simulink model "MCU_vectorControl_with_fieldWeakening_dsPIC33CK_LVMC_FW_Hurst"  (R2018a)
settings: Solver=FixedStepDiscrete  StartTime=0.0  StopTime=10.0  FixedStep=50e-6  RelTol=1e-3  EnableMultiTasking=on
undefined symbols (not defined in the file): A0, A4, AN0, AN1, B0, B2, C12, C13, C14, C7, control, D11, D12, D13, D14, D5, D6, D7, DiscIntNeverNeededParam, inverter, Max, MaxPer, model, ms, NumBits1, NumBits2, P20, P32, P55, P60, P61, P62, P69, P70, P71, P75, P76, P77, P78, Pin, pmsm, PosRange1, PosRange2, PWM1max, Resol, s, Slope1, Slope2, us
libraries: simulink x45, MCHP_Blockset x23
(part 2 of 4)

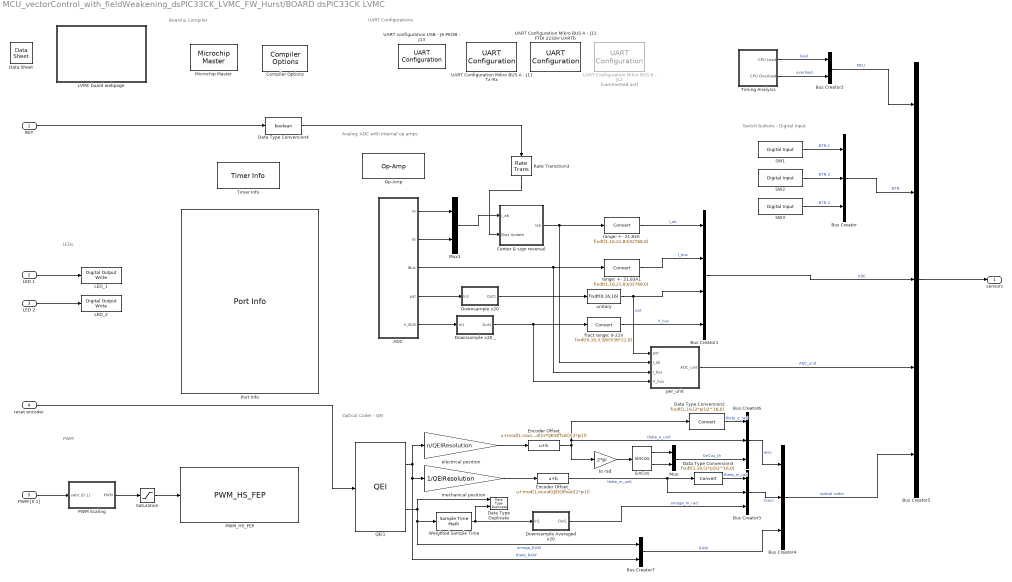
== system MCU_vectorControl_with_fieldWeakening_dsPIC33CK_LVMC_FW_Hurst/BOARD dsPIC33CK LVMC ==
  note: Board & Compiler
  note: Analog: ADC with internal op amps
  note: Optical Coder - QEI
  note: PWM
  note: UART Configurations
  note: LEDs
  note: Switch buttons - Digital Input
  INIT : Inport
  LED 1 : Inport  Port=2
  LED 2 : Inport  Port=3
  reset encoder : Inport  Port=4
  PWM [0 1] : Inport  Port=5  Unit=1
  ADC : Subsystem
  Bus Creator{,3..4,6} (4 alike) : BusCreator  Inputs=3
  Bus Creator1 : BusCreator  Inputs=4
  Bus Creator2 : BusCreator  Inputs=2
  Bus Creator5 : BusCreator  Inputs=5
  Bus Creator7 : BusCreator  Inputs=2
  Center & sign reversal : Subsystem
  Compiler Options : MCHP_Blockset/System Configuration/Compiler Options  Priority=1  LATEST_CMPLR=on  COMP_LIST=Dynamic Options  COMP_LIST_TXT=xc-dsc - v3.10  DFP_LIST=Dynamic Options  DFP_LIST_TXT=from compiler  CMSIS_DSP=Dynamic Options  CMSIS_DSP_TXT=Dynamic Options  USE_64BIT_DOUBLE=off  MCHP_MULTITHREAD_COMPILATION=on  UseCustom_LinkerScript=off  MCHP_MASTERLINK=MCU_vectorControl_with_fieldWeakening_dsPIC33CK_LVMC_FW_Hurst/BOARD dsPIC33CK LVMC/Microchip Master  OPTIMIZATION_LEVEL=2  MPLAB_LINKLIB=relaxed floating-point math  MPLAB_LINKLIB1=default  CodeReplacement=Dynamic Options  CodeReplacement_TXT=Microchip Code Replacement Library for dsPIC  OPTIMIZATION_FLTO=on  OPTIMIZATION_REORDER=off  UNROLL_LOOPS=off  PROCEDURAL_ABSTRACTION=off  GC_SECTIONS=None  MCODE=is more than 32768  MCONST=in code memory  MDATA=Can use all available memory  MSCALAR=Use only memory below address 8192 (faster)  MLARGEARRAY=off  MAGGREGATE=on  HEAP_SIZE=0  OMF=elf  DEBUG_INFO=on  ProduceHexOutput=on  AssemblyListing=off  SaveTemps=off  NO_EDS_WARN=on  PRINT_STATISTICS=off
      settings: SourceProductName=MPLAB Device Blocks for Simulink
  Data Sheet : MCHP_Blockset/System Info/Data Sheet  DOC_Type=datasheet  DOC_MCHP_Id=33FJ64MC802  DOC_FileLastCheckTime=[0 0 0 0 0 0]  cpy_MCHP_Id=33CK256MP508  MCHP_MASTERLINK=MCU_vectorControl_with_fieldWeakening_dsPIC33CK_LVMC_FW_Hurst/BOARD dsPIC33CK LVMC/Microchip Master
      settings: AttributesFormatString=%<cpy_MCHP_Id>  SourceProductName=MPLAB Device Blocks for Simulink
  Data Type Duplicate : DataTypeDuplicate
  Data Type Conversion2 : DataTypeConversion  OutDataTypeStr=fixdt(1,16,(2*pi)/2^16,0)  ConvertRealWorld=Stored Integer (SI)
  Data Type Conversion3 : DataTypeConversion  OutDataTypeStr=fixdt(1,16,(2*pi)/2^16,0)  ConvertRealWorld=Stored Integer (SI)
  Data Type Conversion4 : DataTypeConversion  OutDataTypeStr=boolean
  Downsample Averaged x20 : Subsystem  mask{DownSample=10}
      mask prompts: DownSample "DownSample Factor"
  Downsample x20 : Subsystem  mask{DownSample=20}
      mask prompts: DownSample "DownSample Factor"
  Downsample x20 _ : Subsystem  mask{DownSample=20}
      mask prompts: DownSample "DownSample Factor"
  Encoder Offset : Bias  Bias=mod(1,round((n*QEIOffset)/(2*pi)))
  Encoder Offset_ : Bias  Bias=mod(1,round(QEIOffset/(2*pi)))
  LED_1 : MCHP_Blockset/Digital IO/Digital Output Write  PORT=Dynamic Options  PORT_TXT="E   [ 0 : 15 ]"  PIN=6  PACK=off  SIMULTANEOUS=off  ORDERING=None  SampleTime=-1  MCHP_PORT={Digital Out}{DOU}1:1:E6;  MCHP_MASTERLINK=MCU_vectorControl_with_fieldWeakening_dsPIC33CK_LVMC_FW_Hurst/BOARD dsPIC33CK LVMC/Microchip Master
      settings: SourceProductName=MPLAB Device Blocks for Simulink
  LED_2 : MCHP_Blockset/Digital IO/Digital Output Write  PORT=Dynamic Options  PORT_TXT="E   [ 0 : 15 ]"  PIN=7  PACK=off  SIMULTANEOUS=off  ORDERING=None  SampleTime=-1  MCHP_PORT={Digital Out}{DOU}1:1:E7;  MCHP_MASTERLINK=MCU_vectorControl_with_fieldWeakening_dsPIC33CK_LVMC_FW_Hurst/BOARD dsPIC33CK LVMC/Microchip Master
      settings: SourceProductName=MPLAB Device Blocks for Simulink
  LVMC board webpage : Subsystem
      settings: OpenFcn=|
      | %web('www.microchip.com/DevelopmentTools/ProductDetails.aspx?PartNO=DM330021-2','-browser'); % MCLV2
      | web('https://www.microchip.com/en-us/development-tool/DM330031','-browser'); % LVMC
      | %pause(2);
      | %web('http://www.microchipdirect.com/productsearch.aspx?keywords=AC300020','-browser');
      | %web('www.microchipdirect.com/ProductSearch.aspx?keywords=AC300022','-browser');
      mask Display: image('MCHP_i_Board_LVMC_reduced.jpg');
  Microchip Master : MCHP_Blockset/System Configuration/Microchip Master  Priority=1  PICREF=33CK256MP508  TIMESTEP_REF=PWM1 Trigger 1 + ADC  BUSYFLAG=Dynamic Options  BUSYFLAG_TXT=None  VDD_range=Dynamic Options  PWRTEN=Not used  BOREN=Disable  BODENV=2.7V  BORV=Not used  FPWRT=128ms  DSBOREN=Enable ZPBOR during Deep Sleep Mode  DSLPBOR=Not used  MCLRE=Enabled  SMCLR=MCLR pin generates a normal system Reset  PMDL1WAY=Allow only one reconfiguration  RSTPRI=Device will obtain reset instruction from Primary flash  TEMP=Not used  SOSCSRC=Not used  SOSCSEL=Not used  IOL1WAY=Allow only one reconfiguration  ALTVREF=Not used  DISUVREG=Not used  DSSWEN=Not used  LPCFG=Not used  RTCBAT=Not used  VBTBOR=Not used  WUTSEL=Not used  POWERSAVE=off  ALTI2C=I2C mapped to SDA1/SCL1 pins  ALTI2C1=I2C1 mapped to SDA1/SCL1 pins  ALTI2C2=I2C2 mapped to SDA2/SCL2 pins  ALTI2C3=I2C3 mapped to SDA3/SCL3 pins  FDEVOPT1_ALTI2C1=Primary I2C1 pins are used  FDEVOPT1_ALTI2C2=Primary I2C2 pins are used  FDEVOPT1_SPI2MAPDIS=SPI2 pins are selected by peripheral pin selection feature  ALTQIO=QEA1; QEB1; INDX1 are selected as inputs to QEI1  ALTSS1=SS1A is selected as the I/O pin for SPI1  CMPPOL0=Hysteresis is applied to falling edge  CMPPOL1=Hysteresis is applied to falling edge  FCANIO=Not used  FETHIO=Default Ethernet I/O  FMIIEN=MII Enabled  FSRSSEL=Not used  FUSBIDIO=Controlled by the USB Module  FVBUSONIO=Not used  HPOL=PWM module high side output pins have active-high output polarity  HYST0=45 mV Hysteresis  HYST1=45 mV Hysteresis  I2C1SEL=Not used  LPOL=PWM module low side output pins have active-high output polarity  PWMPIN=PWM module pins controlled by PORT register at device Reset  RTCOSC=Not used  UPLLEN=USB PLL Disabled  UPLLIDIV=Not used  ATMOD8=Not used  ALTPMP=Not used  I2C2SEL=Not used  ALTADREF=Not used  ALTCVREF=Not used  PWMLOCK=PWM registers may be written without key sequence  INT_PRIORITY_DMA=0  MCHP_TIMER_RESULT=[ ]  MCHP_PLLRegisters="[1    100  16387     -1     33]"  MCHPVAR=MCHP.fcy.MIPS=1e+08;MCHP.fcy.SYSCLK=1e+08;MCHP.fcy.ADC=1e+08;MCHP.fcy.Comparator=1e+08;MCHP.fcy.I2C=1e+08;MCHP.fcy.SPI=1e+08;MCHP.fcy.UART=2e+08;MCHP.fcy.Timers=1e+08;MCHP.fcy.OC=1e+08;MCHP.fcy.IC=1e+08;MCHP.fcy.Ports=1e+08;MCHP.fcy.QEI=1e+08;MCHP.fcy.APLL=-1;MCHP.PowerSave=0;MCHP.TimeStepFactor=-20000;MCHP.TimeStep_Timer=-1;MCHP.NTIMERS=1;MCHP.id.name='33CK256MP508';MCHP.id.N=reshape([33 256 508],1,3);MCHP.id.L=reshape({ 'CK','MP',''},1,3);MCHP.id.Arch=3;MCHP.id.maskset='WACG';MCHP.id.dos='02949';MCHP.id.ds='70005349';MCHP.id.archTxt='33xxxx';MCHP.id.clonedfrom='DSPIC33CH128MP508';MCHP.id.isSlave=0;MCHP.id.isMaster=0;MCHP.periph.PPS.reg_RPINRx=reshape([-1 1 1 1 -1 1 1 1 1 1 1 1 1 1 1 1 1 1 1 1 1 1 -1 -1 1 1 1 1 1 1 1 1 1 1 1 1 1 1 1 1 1 1 1 -1 1 1 1 -1 -1 -1 -1 -1 1 -1 1 1 -1 -1 1 1 1 -1 -1 -1 -1 1 1 -1 -1 -1 -1 -1 -1 -1 -1 1 1 -1 -1 -1 -1 -1 -1 -1 1 1 1 1 1 1 1 -1 -1 -1 -1 -1 -1 1 1 1],1,100);MCHP.PPS.dsPIC.RP=reshape([-1 -1 -1 -1 -1 -1 -1 -1 -1 -1 -1 -1 -1 -1 -1 -1 -1 -1 -1 -1 -1 -1 -1 -1 -1 -1 -1 -1 -1 -1 -1 -1 16 17 18 19 20 21 22 23 24 25 26 27 28 29 30 31 32 33 34 35 36 37 38 39 40 41 42 43 44 45 46 47 48 49 50 51 52 53 54 55 56 57 58 59 60 61 62 63],1,80);MCHP.PPS.dsPIC.RPI=reshape(MCHP_Fun.Hex2num('[]'),0,0);MCHP.PPS.dsPIC.RPINR_list=reshape({ '1','INT1','INT2','INT3','5','T1CK','TCKI1','ICM1','TCKI2','ICM2','TCKI3','ICM3','TCKI4','ICM4','TCKI5','ICM5','TCKI6','ICM6','TCKI7','ICM7','TCKI8','ICM8','OCFA','OCFB','PCI8','PCI9','PCI10','PCI11','QEIA1','QEIB1','QEINDX1','QEIHOM1','QEIA2','QEIB2','QEINDX2','QEIHOM2','U1RX','U1DSR','U2RX','U2DSR','SDI1','SCK1_in','SS1_in','REFOI','SDI2','SCK2_in','SS2_in','48','QEIA3','QEIB3','QEINDX3','QEIHOM3','CAN1RX','CAN2RX','U3RX','U3DSR','57','58','SDI3','SCK3_in','SS3_in','CLCINE','CLCINF','CLCING','CLCINH','TCKI9','ICM9','68','69','70','71','72','73','74','OCFC','PCI17','PCI18','78','79','80','81','82','83','84','PCI12','PCI13','PCI14','PCI15','PCI16','SENT1','SENT2','CLCINA','CLCINB','CLCINC','CLCIND','ADCTRG','OCFD','U1CTS','U2CTS','U3CTS'},1,100);MCHP.PPS.dsPIC.RPOR_list=reshape({ '1','U1TX','U1RTS','U2TX','U2RTS','SDO1','SCK1_out','SS1_out','SDO2','SCK2_out','SS2_out','SDO3','SCK3_out','SS3_out','REFCLKO','OCM1','OCM2','OCM3','OCM4','OCM5','OCM6','CAN1TX','CAN2TX','CMP1','CMP2','CMP3','CMP4','U3TX','U3RTS','29','30','31','CMP5','CMP6','PWM4H','PWM4L','PWMEA','PWMEB','QEICCMP1','QEICCMP2','CLC1OUT','CLC2OUT','OCM7','OCM8','PWMEC','PWMED','PTGTRG24','PTGTRG25','SENT1OUT','SENT2OUT','MCCP9A','MCCP9B','MCCP9C','MCCP9D','MCCP9E','MCCP9F','56','57','58','CLC3OUT','CLC4OUT','U1DTR','U2DTR','U3DTR'},1,64);MCHP.PPS.dsPIC.RPV=reshape([176 177 178 179 180 181],1,6);MCHP.PPS.map_RPnR_RPORx=reshape([32 33 34 35 36 37 38 39 40 41 42 43 44 45 46 47 48 49 50 51 52 53 54 55 56 57 58 59 60 61 62 63 64 65 66 67 68 69 70 71 72 73 74 75 76 77 78 79 176 177 178 179 180 181],1,54);MCHP.Rx=reshape([16 34 15 74 2 -1 -1 -1 -1 -1 -1 18 35 28 73 4 -1 -1 -1 -1 -1 -1 20 41 29 72 17 -1 -1 -1 -1 -1 -1 21 43 33 69 19 -1 -1 -1 -1 -1 -1 23 45 63 68 22 -1 -1 -1 -1 -1 -1 -1 55 65 54 24 -1 -1 -1 -1 -1 -1 -1 56 30 53 37 -1 -1 -1 -1 -1 -1 -1 58 40 52 39 -1 -1 -1 -1 -1 -1 -1 60 46 49 42 -1 -1 -1 -1 -1 -1 -1 61 47 48 44 -1 -1 -1 -1 -1 -1 -1 75 66 38 57 -1 -1 -1 -1 -1 -1 -1 76 67 36 59 -1 -1 -1 -1 -1 -1 -1 78 5 27 62 -1 -1 -1 -1 -1 -1 -1 80 6 14 64 -1 -1 -1 -1 -1 -1 -1 1 7 13 77 -1 -1 -1 -1 -1 -1 -1 3 8 10 79 -1 -1 -1 -1 -1 -1],11,16);MCHP.ADC.ANtype=reshape([0 0],1,2);MCHP.ADC.ADCONx=reshape([0 0 0 0 0 0],1,6);MCHP.ADC.ADCHS_0=reshape([0 0],1,2);MCHP.ADC.Flags=reshape([-1 0],1,2);MCHP.ADC.Buffer=reshape([-1 -1],1,2);MCHP.ADC.port=reshape([0 18 23 3 4 16 17 18 19 2 24 25 32 33 34 35 39 38 58 59 64 65 66 67 -1 -1 -1 -1 -1 -1 -1 -1 -1 -1 -1 -1 -1 -1 -1 -1 -1 -1 -1 -1 -1 -1 -1 -1 -1 -1 -1 -1 -1 -1 -1 -1 -1],1,57);MCHP.ADC.port_ALT=reshape([-1 -1 -1 -1],1,4);MCHP.ADC.port_ALTA=reshape([18 1 -1 -1],1,4);MCHP.ADC.port_ALTB=reshape([-1 -1 -1 -1],1,4);MCHP.ADC.port_ALTC=reshape([-1 -1 -1 -1],1,4);MCHP.ADC.port_VrefP=-1;MCHP.ADC.port_VrefM=-1;MCHP.ADC.port_AVdd=-1;MCHP.ADC.port_AVss=-1;MCHP.ADC.ADCDATA=reshape([1 1 1 1 1 1 1 1 1 1 1 1 1 1 1 1 1 1 1 1 1 1 1 1 1 1 0 0 0 0 0 0 0 0 0 0 0 0 0 0 0 0 0 0 0 0 0 0 0 0 0 0 0 0 0 0 0],1,57);MCHP.ADC.HS_SAR.TRGSRC=reshape([1 1 1 1 1 1 1 1 1 1 1 1 1 1 1 1 1 1 1 1 1 1 1 1 1 1 0 0 0 0 0 0],1,32);MCHP.ADC.HS_SAR.nFilters=4;MCHP.ADC.HS_SAR.nDedicatedCore=2;MCHP.ADC.HS_SAR.CALIBRATION=0;MCHP.ADC.HS_SAR.ADCON1L=40960;MCHP.ADC.HS_SAR.ADC_Class3_idxStart=26;MCHP.memory.RAM=24576;MCHP.memory.RAM_XBegin=4096;MCHP.memory.RAM_YBegin=20480;MCHP.memory.RAM_dma=reshape([-1 -1],1,2);MCHP.memory.FLASH_ECC=0;MCHP.DMA.Num=4;MCHP.DMA.CNTmax=65535;MCHP.QEI.QEICONx=reshape([49023 49023 -1 -1 -1 -1],1,6);MCHP.QEI.QEItype=2;MCHP.QEI.Port_QEI_INDX=reshape([-1 -1],1,2);MCHP.QEI.Port_QEI_QEA=reshape([-1 -1],1,2);MCHP.QEI.Port_QEI_QEB=reshape([-1 -1],1,2);MCHP.QEI.Port_QEI_UPDN=reshape([-1 -1],1,2);MCHP.INT.Port=reshape([18 32767 32767 32767 -1],1,5);MCHP.ADC1.port=reshape([-1 -1 -1 -1 -1 -1 -1 -1 -1 -1 -1 -1 -1 -1 -1 -1 -1 -1 -1 -1 -1 -1 -1 -1 -1 -1 -1 -1 -1 -1 -1 -1],1,32);MCHP.ADC2.port=reshape([-1 -1 -1 -1 -1 -1 -1 -1 -1 -1 -1 -1 -1 -1 -1 -1 -1 -1 -1 -1 -1 -1 -1 -1 -1 -1 -1 -1 -1 -1 -1 -1],1,32);MCHP.ADC1N.port=reshape([-1 -1 -1 -1],1,4);MCHP.ADC2N.port=reshape([-1 -1 -1 -1],1,4);MCHP.PWM_HS.Flags=reshape([0 0 0],1,3);MCHP.PWM.port_FLT=reshape([-1 -1 -1 -1 -1 -1 -1 -1 -1 -1 -1 -1 -1 -1 -1 -1 -1 -1 -1 -1 -1 -1 -1 -1 -1 -1 -1 -1 -1 -1 -1 -1 -1],1,33);MCHP.PWM.PWMRef=-1;MCHP.PWM.Flag=0;MCHP.PWM.Port_PWM_l=reshape([31 -1 29 -1 27 -1 48 -1 37 -1 47 -1 43 -1 45 -1 -1 -1 -1 -1 -1 -1 -1 -1],2,12);MCHP.PWM.Port_PWM_h=reshape([30 -1 28 -1 26 -1 49 -1 36 -1 46 -1 42 -1 44 -1 -1 -1 -1 -1 -1 -1 -1 -1],2,12);MCHP.PWM_HS_FEP.nEVTOUT=5;MCHP.IC.Port=reshape([0 0 0 0 0 0 0 0 0 0 0 0 0 0 0 0],1,16);MCHP.IC.type=-1;MCHP.OC.Port=reshape([0 0 0 0 0 0 0 0 0 0 0 0 0 0 0 0],1,16);MCHP.OC.type=-1;MCHP.CN.Port=reshape([-1 -1 -1 -1 -1 -1 -1 -1 -1 -1 -1 -1 -1 -1 -1 -1 -1 -1 -1 -1 -1 -1 -1 -1 -1 -1 -1 -1 -1 -1 -1 -1 -1 -1 -1 -1 -1 -1 -1 -1 -1 -1 -1 -1 -1 -1 -1 -1 -1 -1 -1 -1 -1 -1 -1 -1 -1 -1 -1 -1 -1 -1 -1 -1 -1 -1 -1 -1 -1 -1 -1 -1 -1 -1 -1 -1 -1 -1 -1 -1 -1 -1 -1 -1 -1],1,85);MCHP.CN.PullUp=reshape([31 65535 65535 65535 65535 0 0 0 0 0 0],1,11);MCHP.CN.type=2;MCHP.CN.Flag_PullDown=1;MCHP.SPI.Refs=reshape([1 2 3 0 0 0],1,6);MCHP.SPI.SPIxCON1=-1;MCHP.SPI.SPIxCON2=-1;MCHP.SPI.SPIxFIFOSIZE=4;MCHP.SPI.Port_SDI=reshape([-1 41 -1 -1 -1 -1],1,6);MCHP.SPI.Port_SDO=reshape([-1 56 -1 -1 -1 -1],1,6);MCHP.SPI.Port_SCK=reshape([-1 40 -1 -1 -1 -1],1,6);MCHP.SPI.Port_SS=reshape([-1 -1 -1 -1 -1 -1],1,6);MCHP.I2C.Refs=reshape([1 2 3 0 0],1,5);MCHP.I2C.I2CxCON=49151;MCHP.I2C.NewRegName=2;MCHP.I2C.Port_SDA=reshape([25 21 23 -1 -1],1,5);MCHP.I2C.Port_SCL=reshape([24 22 18 -1 -1],1,5);MCHP.I2C.Port_ASDA=reshape([40 36 52 -1 -1],1,5);MCHP.I2C.Port_ASCL=reshape([41 37 51 -1 -1],1,5);MCHP.I2C.Fuse_Port_SCL_SDA=reshape([29 1 30 1 31 1 -1 -1 -1 -1],2,5);MCHP.I2C.Fuse_Port_ASCL_ASDA=reshape([29 2 30 2 31 2 -1 -1 -1 -1],2,5);MCHP.SCCP.nSCCP=9;MCHP.SCCP.MCCP=reshape([0 0 0 0 0 0 0 0 0],1,9);MCHP.PGA.Port_PGA1P=reshape([-1 -1 -1 -1],1,4);MCHP.PGA.Port_PGA1N=reshape([-1 -1 -1 -1],1,4);MCHP.PGA.Port_PGA2P=reshape([-1 -1 -1 -1],1,4);MCHP.PGA.Port_PGA2N=reshape([-1 -1 -1 -1],1,4);MCHP.PGA.Num=0;MCHP.HS_AnalogComparator.Port_CMP1=reshape([0 33 3 18],1,4);MCHP.HS_AnalogComparator.Port_CMP2=reshape([35 34 59 18],1,4);MCHP.HS_AnalogComparator.Port_CMP3=reshape([23 4 58 18],1,4);MCHP.HS_AnalogComparator.Port_CMP4=reshape([-1 -1 -1 -1],1,4);MCHP.HS_AnalogComparator.PORT_EXTREFx=reshape([-1 -1],1,2);MCHP.HS_AnalogComparator.Port_DACOUTx=reshape([3 -1],1,2);MCHP.HS_AnalogComparator.Num=0;MCHP.Comp.Port_CVrefin=-1;MCHP.Comp.Port_CVref=-1;MCHP.Comp.Port_CVref1O=-1;MCHP.Comp.Port_CVref2O=-1;MCHP.Comp.Port_CxOUT=reshape([32767 32767 32767 32767 32767],1,5);MCHP.Comp.Port_OAxOUT=reshape([0 18 4 -1 -1],1,5);MCHP.Comp.Port_CxINP=reshape([-1 -1 -1 -1 -1],1,5);MCHP.Comp.Port_CxINM=reshape([-1 -1 -1 -1 -1 -1 -1 -1 -1 -1 -1 -1 -1 -1 -1 -1 -1 -1 -1 -1],4,5);MCHP.Comp.Port_OAxINP=reshape([2 20 34 -1 -1],1,5);MCHP.Comp.Port_OAxINM=reshape([1 19 33 -1 -1],1,5);MCHP.Comp.nComp=reshape([5 0 0],1,3);MCHP.Comp.OpAmp=0;MCHP.Comp.CVRCON=reshape([0 0],1,2);MCHP.Comp.CMCON=0;MCHP.CDAC.Port_DACx=reshape([-1 -1 -1],1,3);MCHP.CDAC.nCDAC=0;MCHP.UART.port_Rx=reshape([32767 32767 32767 -1 -1 -1],1,6);MCHP.UART.port_Tx=reshape([32767 32767 32767 -1 -1 -1],1,6);MCHP.UART.port_ARx=reshape([-1 -1],1,2);MCHP.UART.port_ATx=reshape([-1 -1],1,2);MCHP.UART.port_RTS=reshape([32767 32767 32767 -1 -1 -1],1,6);MCHP.UART.port_CTS=reshape([32767 32767 32767 -1 -1 -1],1,6);MCHP.UART.reg_UxMODE=reshape([48127 48127 48127 -1 -1 -1],1,6);MCHP.UART.reg_UxSTA=reshape([65535 65535 65535 -1 -1 -1],1,6);MCHP.modsrc.DOS_04094_cpu_33a_v1_dspic33a=0;MCHP.modsrc.DOS_04436_perseus_dspic33a=0;MCHP.modsrc.DOS_04928_gpio_ports_upb_v2_dspic33a=0;MCHP.modsrc.DOS_02672_math_progcrc_upb_v1_dspic33a=0;MCHP.modsrc.DOS_04993_sec_32bit_cp_upb_v1_dspic33a=0;MCHP.modsrc.DOS_03681_bmx_33a_upb_v1_dspic33a=0;MCHP.modsrc.DOS_03459_adc_pc_ctrl_upb_v2_dspic33a=0;MCHP.modsrc.DOS_04302_pwm_pc_upb_v3_dspic33a=0;MCHP.modsrc.DOS_03076_uart_protocol_upb_v1_dspic33a=0;MCHP.modsrc.DOS_01482_spi_i2s_upb_v1_dspic33a=0;MCHP.modsrc.DOS_05155_i2c_upb_v4_dspic33a=0;MCHP.modsrc.DOS_02359_sent_j2716_upb_v1_dspic33a=0;MCHP.modsrc.DOS_05177_qei_32b_upb_v2_dspic33a=0;MCHP.modsrc.DOS_01512_ccp_mccp_upb_v1_dspic33a=0;MCHP.modsrc.DOS_03496_dac_pdm_nbit_upb_v2_dspic33a=0;MCHP.modsrc.DOS_02673_tmr_classa_upb_v1_dspic33a=0;MCHP.modsrc.DOS_04776_perf_mon_upb_v1_dspic33a=0;MCHP.modsrc.DOS_03680_pfm_pbu_33a_upb_v1_dspic33a=0;MCHP.modsrc.DOS_04649_sec_pac_upb_v0_dspic33a=0;MCHP.modsrc.DOS_03966_io_integrity_monitor_upb_v1_dspic33a=0;MCHP.modsrc.DOS_04641_biss_master_upb_v1_dspic33a=0;MCHP.modsrc.DOS_04077_dma_upb_v1_dspic33a=0;MCHP.modsrc.DOS_04549_nvm_ctrl_32bit_upb_v1_dspic33a=0;MCHP.modsrc.DOS_04449_clk_cru_33a_upb_v1_dspic33a=0;MCHP.modsrc.DOS_03850_clk_monitor_upb_v1_dspic33a=0;MCHP.modsrc.DOS_04342_osc_rc8mhz_ctrl_upb_v4_dspic33a=0;MCHP.modsrc.DOS_04650_wdt_upb_v4_dspic33a=0;MCHP.modsrc.DOS_05178_ptg_pc_upb_v1_dspic33a=0;MCHP.modsrc.DOS_04181_data_ram_ctrl_upb_v1_dspic33a=0;MCHP.modsrc.DOS_04735_wdt_dmt_upb_v6_dspic33a=0;MCHP.modsrc.DOS_01577_cla_clc_upb_v1_dspic33a=0;MCHP.modsrc.DOS_03516_pwr_sib_upb_v3_dspic33a=0;MCHP.modsrc.DOS_03495_amp_pad_opamp_ctrl_upb_v2_dspic33a=0;MCHP.modsrc.DOS_05308_pegasus_dspic33a=0;MCHP.modsrc.DOS_02976_adc_12b_upb_v2_dspic33a=0;MCHP.modsrc.DOS_05404_adc_pc_ctrl_upb_v3_dspic33a=0;MCHP.modsrc.DOS_05226_pwm_pc_upb_v4_dspic33a=0;MCHP.modsrc.DOS_05226_apwm_pc_upb_v4_dspic33a=0;MCHP.modsrc.DOS_05431_dac_pdm_nbit_upb_v3_dspic33a=0;MCHP.modsrc.DOS_04649_sec_pac_upb_v1_dspic33a=0;MCHP.modsrc.DOS_05461_pwr_sib_upb_v4_dspic33a=0;MCHP.modsrc.DOS_05420_amp_vref_ctl_upb_v1_dspic33a=0;MCHP.modsrc.DOS_03267_adc_soft_code_seq_v1_dspic33a=0;MCHP.modsrc.DOS_04537_can_fd_upb_v3_dspic33a=0;MCHP.modsrc.DOS_05346_sec_cam_lite_v2_dspic33a=0;MCHP.modsrc.DOS_02551_cpu_16bit_v7=1;MCHP.modsrc.DOS_01520_wdt_dmt_upb_v1_16bit=1;MCHP.modsrc.DOS_02359a_sent_j2716_upb_v1=1;MCHP.modsrc.DOS_02672_math_progcrc_upb_v1_16bit=1;MCHP.modsrc.DOS_01577_cla_clc_upb_v1=1;MCHP.modsrc.DOS_02915_ecc_v2=1;MCHP.modsrc.DOS_02673_tmr_classa_upb_v1_16bit=1;MCHP.modsrc.DOS_01494_qei_32b_upb_v1_16bit=1;MCHP.modsrc.DOS_02472_ppi_pmp16_upb_v1_16bit=1;MCHP.modsrc.DOS_01441_i2c_upb_v1_16bit_TLAH=1;MCHP.modsrc.DOS_03076_uart_protocol_upb_v1_16bit=1;MCHP.modsrc.DOS_01482=1;MCHP.modsrc.DOS_01483_pwm_16bit=1;MCHP.modsrc.DOS_03247_CAN_FD_UPB_V2_16_bit=1;MCHP.modsrc.DOS_02949_WACG=1;MCHP.modsrc.DOS_02316_nvm_ctrl_v1_16bit=1;MCHP.modsrc.DOS_03349_amp_pad_opamp_ctrl_upb_v1=1;MCHP.modsrc.DOS_02653_afe_current_bias_ctrl_upb_v1_16bit=1;MCHP.modsrc.DOS_01459_ptg_pc_upb_v1_16bit=1;MCHP.modsrc.DOS_01512_ccp_mccp_upb_v1_16bit=1;MCHP.modsrc.DOS_02519_dma_sfr_16bit_v2=1;MCHP.modsrc.DOS_02508c11=1;MCHP.modsrc.DOS_02475_dac_pdm_nbit_upb_v1_16bit=1;MCHP.modsrc.DOS_02467_gpio_upb_v1_16bit=1;MCHP.modsrc.DOS_00805_rst_integration_v4=1;MCHP.modsrc.DOS_02659_clk_sib_v12=1;MCHP.modsrc.DOS_02237_osc_dco_ctrl_upb_v1_16bit=1;MCHP.modsrc.DOS_02674_wdt_upb_v1_16bit=1;MCHP.modsrc.DOS_01407=1;MCHP.modsrc.DOS_03994_WAC07=0;MCHP.modsrc.DOS_02552_msi_upb_v1_Master=0;MCHP.modsrc.DOS_03667_pwm_pc_upb_v2_16bit=0;MCHP.modsrc.DOS_04180_drm_ctrl_ecc_v1=0;MCHP.modsrc.DOS_03431_STX03=0;MCHP.modsrc.DOS_03516_pwr_sib_upb_v3=0;MCHP.modsrc.DOS_02552_msi_upb_v1_Slave=0;MCHP.modsrc.DOS_04621_amp_pga_ctrl_upb_v3=0;MCHP.modsrc.DOS_02497_WACV=0;MCHP.modsrc.DOS_02593_amp_pga_ctrl_pb_v2_16bit=0;MCHP.modsrc.DOS_01461_afe_ctmu_con_upb_v1_16bit=0;MCHP.modsrc.DOS_02497_WACA=0;MCHP.modsrc.DOS_02478_uart_irda_upb_v1_16bit=0;MCHP.modsrc.DOS_00929=0;MCHP.modsrc.DOS_01198=0;MCHP.modsrc.DOS_03029_WACH=0;MCHP.modsrc.DOS_01483_apwm_16bit=0;MCHP.modsrc.DOS_04797_WAC0A=0;MCHP.modsrc.DOS_04884_WAC0B=0;MCHP.modsrc.DOS_04797_WAC09=0;MCHP.modsrc.DOS_03662_WACU=0;MCHP.modsrc.DOS_00794=0;MCHP.modsrc.DOS_00931=0;MCHP.modsrc.DOS_00932=0;MCHP.modsrc.DOS_00942=0;MCHP.modsrc.DOS_00938=0;MCHP.modsrc.DOS_00996=0;MCHP.modsrc.DOS_00997=0;MCHP.modsrc.DOS_00998=0;MCHP.modsrc.DOS_00209=0;MCHP.modsrc.DOS_01555_adc=0;MCHP.modsrc.DOS_01293=0;MCHP.modsrc.DOS_00828=0;MCHP.modsrc.DOS_01116=0;MCHP.modsrc.DOS_01017_RPORx=0;MCHP.modsrc.DOS_01017_RPINRx=0;MCHP.modsrc.DOS_01555_nvm_tsmc18_v2_16bit=0;MCHP.modsrc.DOS_00804=0;MCHP.modsrc.DOS_00826=0;MCHP.modsrc.DOS_01555_TLAK_PMDx=0;MCHP.modsrc.DOS_01555_TLAK_INT_=0;MCHP.modsrc.DOS_00933=0;MCHP.modsrc.DOS_01555=0;MCHP.modsrc.DOS_01555_ptg=0;MCHP.modsrc.DOS_00958=0;MCHP.modsrc.DOS_01117_PORTx=0;MCHP.modsrc.DOS_00999=0;MCHP.modsrc.DOS_01041=0;MCHP.modsrc.DOS_00892=0;MCHP.modsrc.DOS_01287_TLAC_PMDx=0;MCHP.modsrc.DOS_01287_TLAC_INT_=0;MCHP.modsrc.DOS_01424=0;MCHP.modsrc.DOS_01332=0;MCHP.modsrc.DOS_01468_PMBA_current_source=0;MCHP.modsrc.DOS_02291_PGA=0;MCHP.modsrc.DOS_01467_Comparator=0;MCHP.modsrc.DOS_01498_TLAY=0;MCHP.modsrc.DOS_00993_PLL_120MHz=0;MCHP.modsrc.DOS_01332_ptg_pc_v1=0;MCHP.modsrc.DOS_00958_pwm_TLAY=0;MCHP.modsrc.TLAY_IOPorts=0;MCHP.modsrc.DOS_00929q=0;MCHP.modsrc.DOS_02415_spi_v5=0;MCHP.modsrc.DOS_RPINRx_16bit_2=0;MCHP.modsrc.DOS_01497_TLAH_PMDx=0;MCHP.modsrc.DOS_02550_TLAL_INT=0;MCHP.modsrc.DOS_00958_pwm_TLAH=0;MCHP.modsrc.DOS_01287_TLAH_INT_=0;MCHP.modsrc.DOS_01113=0;MCHP.modsrc.DOS_01017_PMDx=0;MCHP.modsrc.DOS_00927=0;MCHP.modsrc.DOS_01080=0;MCHP.modsrc.DOS_00794_cpu_16bit_v3=0;MCHP.modsrc.DOS_02192_TLCD_PMDx=0;MCHP.modsrc.DOS_02192_TLCD_INT_=0;MCHP.modsrc.DOS_02192_cmp=0;MCHP.modsrc.DOS_00958_pwm_TLCD=0;MCHP.modsrc.DOS_02192_PORTx_TLCD=0;MCHP.modsrc.DOS_00936=0;MCHP.modsrc.DOS_00995=0;MCHP.modsrc.DOS_00546=0;MCHP.modsrc.DOS_00474=0;MCHP.modsrc.DOS_02481_WACK_MC_Config=0;MCHP.modsrc.DOS_03088_pfm_cache_ocp_v2_WACK=0;MCHP.modsrc.DOS_02819_pfm_ctrl_32bit_upb_v2=0;MCHP.modsrc.DOS_02674_wdt_upb_v1_32bit=0;MCHP.modsrc.DOS_01520_wdt_dmt_upb_v1=0;MCHP.modsrc.DOS_02869_icd_jtag_bvci_upb_v2=0;MCHP.modsrc.DOS_02823_WACJ_clk_cru_upb_v2=0;MCHP.modsrc.DOS_02823_WACN_clk_cru_upb_v2=0;MCHP.modsrc.DOS_01423_RPINRx=0;MCHP.modsrc.DOS_02481_RPORx=0;MCHP.modsrc.DOS_02511_pwr_sib_upb_v1_32bit=0;MCHP.modsrc.DOS_02907_WACN_GP_int_evic_v3=0;MCHP.modsrc.DOS_01500_dma_bvci_v2=0;MCHP.modsrc.DOS_02141_tmr_classa_pb_v2=0;MCHP.modsrc.DOS_02815_tmr_classb_upb_v1=0;MCHP.modsrc.DOS_00740_icap_pb_v1=0;MCHP.modsrc.DOS_00749_ocmp_pb_v1=0;MCHP.modsrc.DOS_01441_i2c_upb_v1_32bit=0;MCHP.modsrc.DOS_01329_spi_pb_v2=0;MCHP.modsrc.DOS_02478_uart_irda_upb_v1_32bit=0;MCHP.modsrc.DOS_03554_cmp_control_upb_v2_32bit=0;MCHP.modsrc.DOS_01445_dac_nbit__control_upb_v1_32bit=0;MCHP.modsrc.DOS_01461_afe_ctmu_con_upb_v1=0;MCHP.modsrc.DOS_01577_cla_clc_upb_v1_32bit=0;MCHP.modsrc.DOS_02467_gpio_ports_upb_v1=0;MCHP.modsrc.DOS_02508_adc_sar_ctrl_upb_v1_PIC32MK=0;MCHP.modsrc.DOS_01261_tmr_rtcc_pb_v2=0;MCHP.modsrc.DOS_01475_lpwr_deep_sleep_ctrl_v2=0;MCHP.modsrc.DOS_EIP_00136_ssx_v1=0;MCHP.modsrc.DOS_02907_WACN_MC_int_evic_v3=0;MCHP.modsrc.DOS_01477_pwm_mc_upb_v1=0;MCHP.modsrc.DOS_01494_qei_32b_upb_v1=0;MCHP.modsrc.DOS_03247_can_fd_upb_v2_pic32mk=0;MCHP.modsrc.DOS_02907_WACK_MC_int_evic_v3=0;MCHP.modsrc.DOS_02514_dfm_strl_sst_upb_v1=0;MCHP.modsrc.DOS_02472_ppi_pmp16_upb_v1=0;MCHP.modsrc.DOS_02813a_usb_otgcore_pb_v3=0;MCHP.modsrc.DOS_02481_WACJ_MC_Config=0;MCHP.modsrc.DOS_02569_pfm_cache_ocp_v1=0;MCHP.modsrc.DOS_02481_WACJ_MC_int_evic_v3=0;MCHP.modsrc.DOS_01459_ptg_pc_upb_v1_SIC=0;MCHP.modsrc.DOS_01427_cmp_control_upb_v1_32bit=0;MCHP.modsrc.DOS_01152_can_bvci_v1=0;MCHP.modsrc.DOS_02787_WACD_Config=0;MCHP.modsrc.DOS_00800_dac_4bit_ctrl_pb_v1=0;MCHP.modsrc.DOS_01539_icd_jtag_pb_v2=0;MCHP.modsrc.DOS_02823_clk_cru_upb_v2=0;MCHP.modsrc.DOS_01423_RPORx=0;MCHP.modsrc.DOS_02907_WACD_int_evic_v3=0;MCHP.modsrc.DOS_00734_uart_irda_pb_v1=0;MCHP.modsrc.DOS_00687_tmr_classa_pb_v1=0;MCHP.modsrc.DOS_00745_tmr_classb_pb_v1=0;MCHP.modsrc.DOS_02508_adc_sar_ctrl_upb_v1=0;MCHP.modsrc.DOS_00866_cmp_control_pb_v2=0;MCHP.modsrc.DOS_01114_eth_bvci_v1=0;MCHP.modsrc.DOS_02831_usb_clk_rst_v2=0;MCHP.modsrc.DOS_01643_pfm_cache_ahb_v2=0;MCHP.modsrc.DOS_EIP_00206r5_sqi_v2=0;MCHP.modsrc.DOS_EIP_00124_usb_hs_otgcore_v1=0;MCHP.modsrc.DOS_EIP_00218_math_rng_ahbs_v2=0;MCHP.modsrc.DOS_EIP_00109_ebi_v1=0;MCHP.modsrc.DOS_EIP_00158_crypto_v1=0;MCHP.PortBase=16;MCHP.PortPrefixe='P';MCHP.clock.PBxDIV=-1;MCHP.clock.CLKx_INTDIV=reshape([-1 -1 -1 -1 -1 -1 -1 -1 -1 -1 -1 -1 -1],1,13);MCHP.clock.CLKx_FRACDIV=reshape([-1 -1 -1 -1 -1 -1 -1 -1 -1 -1 -1 -1 -1],1,13);  MCHP_CRC=19007516  BTMODE=Device is in Single Boot (legacy) mode  RES1=Not used  RES2=Not used  ALTCMPI=Not used  BOREN1=Not used  ALTRB6=Not used  WDTEN=Disable  DBCC=No Cross Connection between DAC outputs  BOREN0=Enabled  DMTIVT=Not used  DMTCNT=2^31 (2147483648)  DMTEN=Dead Man Timer is Disabled and can be enabled by software  ON=Not used  USERID=Not used  RESERVED1=Not used  DMTINTV=Window/Interval value is 127/128 counter value  WDTSPGM=WDT stops during Flash programming  FDMTEN=Deadman Timer is disabled  BOOTISA=Boot code and Exception code is MIPS32  FSLEEP=Flash is powered down when the device is in Sleep mode  TSEQ=Not used  CSEQ=Not used  BORLVL=BOR trip point is 2.96 V  BSSO=Normal startup operation after reset; execute instruction at 0x000000  MCA=Flash read accesses are 2 cycle to support maximum processor frequency of operation  MAXTEMP=20 ns flash access  CFGAN14=Device pin is input to AN14  CFGAN15=Device pin is input to AN15  BISTDIS=mBIST on reset feature disabled  NOBTSWP=BOOTSWP instruction is disabled  BSEQ=Not used  IBSEQ=Not used  SMB3EN=SMBus 3.0 input levels  FUSBIDIO2=USBID pin is controlled by the USB2 module  FVBUSIO2=VBUSON pin is controlled by the USB2 module  FUSBIDIO1=USBID pin is controlled by the USB1 module  FVBUSIO1=VBUSON pin is controlled by the USB1 module  VBATBOREN=Enable ZPBOR during VBAT Mode  FDSEN=Enable DSEN bit in DSCON  BORSEL=BOR trip voltage 2.1v (Non-OPAMP deviced operation)  POSCFGAIN=Gain is G3  POSCAGCDLY=Settling time = 25ms x AGCRNG  POSCAGCRNG=Range 1x  POSCAGC=Automatic Gain Control for Oscillator  FDBGWP=Not used  FNOSC=Internal Fast RC (FRC)  FPR=ECIO w/ PLL 16x  FOSFPR=HS3 w/PLL 16x  FOS=Primary Oscillator  FRANGE=High Range  OSCILLATOR_SELECT=Internal Fast RC (FRC)  OSCILLATOR_SELECT_spd=Internal Fast RC (FRC)  QUARTZ=8e6  QUARTZ_spd=8e6  POSCGAIN=2x gain setting  POSCBOOST=Boost the kick start of the oscillator  SOSCGAIN=2x gain setting  SOSCBOOST=Boost the kick start of the oscillator  ACTIV_PLL=on  ACTIV_PLL_spd=on  MIPS_DESIRED=100e6  MIPS_DESIRED_spd=100e6  CPUDIV=Divide by 1  FPLLMUL=Not used  FPLLIDIV=8x Divider  POSCFREQ=Not used  POSCMD=Primary Oscillator Disabled  POSCMOD=Primary Oscillator Disabled  MIPS=100 * 1e6  ACLKCON=Optimized for PWM resolution & ADC conversion speed  ACLKCON_spd=Optimized for PWM resolution & ADC conversion speed  FPLLODIV=32x Divider  PLLKEN=PLL lock signal will be used to disable PLL clock output if lock is lost  FCKSM=Clock switching is enabled;Fail-safe Clock Monitor is disabled  FCKSMEN=Sw Disabled; Mon Disabled  IESO=Start up with FRC; then switch  DSWDTPS=1:2^36  FWDTEN=WDT controlled via SW; use WDTCON.ON bit  FWDTWINSZ=Window size is 25%  FWPSA=1:512  FWPSA0=1:128  FWPSB=1:16  WDT=Disable  WDTPOST=1:32768  WDTPRE=1:128  WDTPS=1:32768  WINDIS=Watchdog Timer operates in Non-Window mode  WWDTEN=Non-Window mode  DSWDTEN=Enable DSWDT during Deep Sleep Mode  DSWDTOSC=Select LPRC as DSWDT Reference clock  FWDT_RCLKSEL=WDT Run Mode uses BFRC:256  FWDT_RWDTPS=1:2147483648  FWDT_SWDTMPS=1:2147483648  FWDT_WDTEN=WDT is controlled by software; use WDTCON.ON bit  FWDT_WDTRSTEN=WDT event generates a reset  FWDT_WDTWIN=WDT Window is 25% of WDT period  FWDT_WINEN=Watchdog Timer operates in Window mode  FPBDIV=Not used  FSOSCEN=Disable Secondary Oscillator  LPRCSEL=Not used  OSCIOFCN=Not used  OSCIOFNC=general purpose digital I/O pin  LVRCFG=Not used  PLL_96MHZ=Not used  PLL96MHZ=Not used  PLLDIV=Not used  WDTCLK=Not used  WDTCMX=Not used  WDTWIN=WDT Window is 25% of WDT period  XTCFG=24-32 MHz crystals  XTBST=Boost the kick-start  PLLSS=Not used  FPLLRNG=34-68 MHz Input  FPLLICLK=FRC is input to the System PLL  FPLLMULT=PLL Multiply by 128  UPLLFSEL=USB PLL input is 24 MHz  APL=Aux Flash Code protect is disabled  APLK=Aux Flash Write Protection or Code Protection is Enabled  AWRP=Auxiliary program memory is not write-protected  BSS=No Protection (other than BWRP)  BWP=Not used  BWRP=Boot Segment may be written  CP=Protection Disabled  EBS=No Boot EEPROM  ESS=No Segment Data EEPROM  GCP=General Segment Code protect is Disabled  GSS=No Protection (other than GWRP)  GSS0=Not used  GSSK=General Segment Write Protection or Code Protection is Enabled  GWRP=General Segment may be written  PWP=Not used  RBS=No Boot RAM  RSS=No Secure RAM  SSS=No Secure Segment  SWRP=Secure segment may be written  WPCFG=Not used  WPDIS=Not used  WPEND=Not used  WPFP=Not used  DFMCY=Not used  BSS2=No Boot Segment  BSEN=No Boot Segment  CWRP=Configuration Segment may be written  CSS=No Protection (other than CWRP)  AIVTDIS=Disabled AIVT  BSLIM=Not used  BTSWP=BOOTSWP instruction is disabled  CTXT1=Not Assigned  CTXT2=Not Assigned  SEQNUM=Not used  nSEQNUM=Not used  PGL1WAY=Allow only one reconfiguration  FECCCON=ECC and Dynamic ECC are disabled (ECCCON bits are writable)  EXTDDRSIZE=Not used  ICESEL=Communicate on PGEC1/PGED1  ICS=Communicate on PGC3 and PGD3  JTAGEN=Disable  FICD_JTAGEN=Disable  COE=Not used  RES=Not used  DEBUG=Debugger is disabled  BACKBUG=Not used  BKBUG=Not used  RETCFG=Not used  TRCEN=Trace features in the CPU are enabled  DBGPER=Allow CPU access to all permission regions  EJTAGBEN=Normal EJTAG functionality  S1ICS=Communicate on PGC3 and PGD3  S1ISOLAT=The Secondary can operate (in debug mode) even if the SLVEN bit in the MSI is zero  RWDTPS=1:1048576  RCLKSEL=Always use LPRC  SWDTPS=1:1048576  DMTIVTL=Not used  DMTIVTH=Not used  DMTCNTL=Not used  DMTCNTH=Not used  DMTDIS=Dead Man Timer is Disabled and can be enabled by software  SMBEN=SMBus input threshold is enabled  SPI2PIN=SPI2 uses I/O remap (PPS) pins  CTXT3=Not Assigned  CTXT4=Not Assigned  MBXM0=Mailbox register configured for Main data read (Secondary to Main data transfer)  MBXM1=Mailbox register configured for Main data read (Secondary to Main data transfer)  MBXM2=Mailbox register configured for Main data read (Secondary to Main data transfer)  MBXM3=Mailbox register configured for Main data read (Secondary to Main data transfer)  MBXM4=Mailbox register configured for Main data read (Secondary to Main data transfer)  MBXM5=Mailbox register configured for Main data read (Secondary to Main data transfer)  MBXM6=Mailbox register configured for Main data read (Secondary to Main data transfer)  MBXM7=Mailbox register configured for Main data read (Secondary to Main data transfer)  MBXM8=Mailbox register configured for Main data read (Secondary to Main data transfer)  MBXM9=Mailbox register configured for Main data read (Secondary to Main data transfer)  MBXM10=Mailbox register configured for Main data read (Secondary to Main data transfer)  MBXM11=Mailbox register configured for Main data read (Secondary to Main data transfer)  MBXM12=Mailbox register configured for Main data read (Secondary to Main data transfer)  MBXM13=Mailbox register configured for Main data read (Secondary to Main data transfer)  MBXM14=Mailbox register configured for Main data read (Secondary to Main data transfer)  MBXM15=Mailbox register configured for Main data read (Secondary to Main data transfer)  MBXHSA=MSIxMBXD15 assigned to mailbox handshake protocol block A  MBXHSB=MSIxMBXD15 assigned to mailbox handshake protocol block B  MBXHSC=MSIxMBXD15 assigned to mailbox handshake protocol block C  MBXHSD=MSIxMBXD15 assigned to mailbox handshake protocol block D  MBXHSE=MSIxMBXD15 assigned to mailbox handshake protocol block E  MBXHSF=MSIxMBXD15 assigned to mailbox handshake protocol block F  MBXHSG=MSIxMBXD15 assigned to mailbox handshake protocol block G  MBXHSH=MSIxMBXD15 assigned to mailbox handshake protocol block H  HSAEN=Mailbox data flow control handshake protocol block disabled  HSBEN=Mailbox data flow control handshake protocol block disabled  HSCEN=Mailbox data flow control handshake protocol block disabled  HSDEN=Mailbox data flow control handshake protocol block disabled  HSEEN=Mailbox data flow control handshake protocol block disabled  HSFEN=Mailbox data flow control handshake protocol block disabled  HSGEN=Mailbox data flow control handshake protocol block disabled  HSHEN=Mailbox data flow control handshake protocol block disabled  CPRA0=Main core owns pin  CPRA1=Main core owns pin  CPRA2=Main core owns pin  CPRA3=Main core owns pin  CPRA4=Main core owns pin  CPRB0=Main core owns pin  CPRB1=Main core owns pin  CPRB2=Main core owns pin  CPRB3=Main core owns pin  CPRB4=Main core owns pin  CPRB5=Main core owns pin  CPRB6=Main core owns pin  CPRB7=Main core owns pin  CPRB8=Main core owns pin  CPRB9=Main core owns pin  CPRB10=Main core owns pin  CPRB11=Main core owns pin  CPRB12=Main core owns pin  CPRB13=Main core owns pin  CPRB14=Main core owns pin  CPRB15=Main core owns pin  CPRC0=Main core owns pin  CPRC1=Main core owns pin  CPRC2=Main core owns pin  CPRC3=Main core owns pin  CPRC4=Main core owns pin  CPRC5=Main core owns pin  CPRC6=Main core owns pin  CPRC7=Main core owns pin  CPRC8=Main core owns pin  CPRC9=Main core owns pin  CPRC10=Main core owns pin  CPRC11=Main core owns pin  CPRC12=Main core owns pin  CPRC13=Main core owns pin  CPRC14=Main core owns pin  CPRC15=Main core owns pin  CPRD0=Main core owns pin  CPRD1=Main core owns pin  CPRD2=Main core owns pin  CPRD3=Main core owns pin  CPRD4=Main core owns pin  CPRD5=Main core owns pin  CPRD6=Main core owns pin  CPRD7=Main core owns pin  CPRD8=Main core owns pin  CPRD9=Main core owns pin  CPRD10=Main core owns pin  CPRD11=Main core owns pin  CPRD12=Main core owns pin  CPRD13=Main core owns pin  CPRD14=Main core owns pin  CPRD15=Main core owns pin  CPRE0=Main core owns pin  CPRE1=Main core owns pin  CPRE2=Main core owns pin  CPRE3=Main core owns pin  CPRE4=Main core owns pin  CPRE5=Main core owns pin  CPRE6=Main core owns pin  CPRE7=Main core owns pin  CPRE8=Main core owns pin  CPRE9=Main core owns pin  CPRE10=Main core owns pin  CPRE11=Main core owns pin  CPRE12=Main core owns pin  CPRE13=Main core owns pin  CPRE14=Main core owns pin  CPRE15=Main core owns pin  S1FNOSC=Internal Fast RC (FRC) Oscillator with postscaler  S1IESO=Start up with FRC; then switch  S1OSCIOFNC=OSC2 is clock output  S1FCKSM=Both Clock switching and Fail-safe Clock Monitor are disabled  S1PLLKEN=S1PLLKEN_ON  S1RWDTPS=1:1048576  S1RCLKSEL=Always use LPRC  S1WINDIS=Watchdog Timer operates in Non-Window mode  S1WDTWIN=WDT Window is 25% of WDT period  S1SWDTPS=1:1048576  S1FWDTEN=use WDTCON.ON bit  S1DEBUG=Not used  S1NOBTSWP=BOOTSWP instruction is disabled  S1ALTI2C1=I2C1 mapped to SDA1/SCL1 pins  S1SPI1PIN=Secondary SPI1 uses I/O remap (PPS) pins  S1SSRE=Secondary generated resets will reset the Secondary Enable Bit in the MSI module  S1MSRE=The Main software oriented RESET events (RESET Op-Code; Watchdog timeout; TRAP reset; illegalInstruction) will also cause the Secondary subsystem to reset  S1CTXT1=Not Assigned  S1CTXT2=Not Assigned  S1CTXT3=Not Assigned  S1CTXT4=Not Assigned  S1IOL1WAY=Allow only one reconfiguration  S1BSSO=Normal startup operation after reset; execute instruction at 0x000000  S1BACKBUG=Not used  S1BISTDIS=Secondary BIST on reset feature disabled  S1DMTIVTL=Not used  S1DMTIVTH=Not used  S1DMTCNTL=Not used  S1DMTCNTH=Not used  S1DMTDIS=Secondary Dead Man Timer is Disabled and can be enabled by software
      settings: SourceProductName=MPLAB Device Blocks for Simulink
  Mux : Mux  Inputs=2
  Mux1 : Mux  Inputs=2
  Op-Amp : MCHP_Blockset/Analog IO/Op-Amp  Priority=-2000  OpAmp1=Enabled with positive and negative inputs  OpAmp2=Enabled with positive and negative inputs  OpAmp3=Enabled with positive and negative inputs  S_INPUT=[-1]  S_INPUT_Size=[3]  S_OUTPUT=[]  S_OUTPUT_Size=[]  S_ListCustomDatatype=S.S_ListCustomDatatype={};  MCHP_USER_INTERRUPTS=0  MCHP_PORT={OA1 Output}{OA1out}14:2:A0;{OA1 IN+}{OA1in+}14:2:A2;{OA1 IN-}{OA1in-}14:2:A1;{OA2 Output}{OA2out}14:2:B2;{OA2 IN+}{OA2in+}14:2:B4;{OA2 IN-}{OA2in-}14:2:B3;{OA3 Output}{OA3out}14:2:A4;{OA3 IN+}{OA3in+}14:2:C2;{OA3 IN-}{OA3in-}14:2:C1;  MCHP_MASTERLINK=MCU_vectorControl_with_fieldWeakening_dsPIC33CK_LVMC_FW_Hurst/BOARD dsPIC33CK LVMC/Microchip Master  MCHP_CRC=717193
      settings: SourceProductName=MPLAB Device Blocks for Simulink
  PWM Scaling : Subsystem
  PWM_HS_FEP : MCHP_Blockset/PWM IO/PWM_HS_FEP  Priority=-2000  PWMx_MODSEL=Center Aligned  PWMx_CLKSEL=no scaling  PWM_ClockResolution_DIVSEL=Dynamic Options  PWM_ClockResolution_DIVSEL_TXT=auto  PWM_ClockResolution_FSCL=Dynamic Options  PWM_ClockResolution_FSCL_TXT=auto - best resolution  PWM_ClockResolution_NoScaling=Dynamic Options  PWM_ClockResolution_NoScaling_TXT="Resol: 0.005208(us)  -  MaxPer: 0.000341(s)"  MaxPeriod_s=50e-6  InitPeriode_s=50e-6  InitDutyCycleP_s=25e-6  InitDutyCycleS_s=10e-6  InitPhase_s=-1  evalin_ws=PWM1max=MCHP_Fun.Hex2num('40B3880000000000');PWM2max=MCHP_Fun.Hex2num('40B3880000000000');PWM4max=MCHP_Fun.Hex2num('40B3880000000000');  SampleTime=-1  S_INPUT=[-1]  S_INPUT_Size=[3]  S_OUTPUT=[]  S_OUTPUT_Size=[]  S_ListCustomDatatype=S.S_ListCustomDatatype={};  MCHP_USER_INTERRUPTS=0  MCHP_PORT={PWMH1 }{PWMH1}32:4:B14;{PWMH2 }{PWMH2}32:4:B12;{PWMH4 }{PWMH4}32:4:D1;{PWML1}{PWML1}32:4:B15;{PWML2}{PWML2}32:4:B13;{PWML4}{PWML4}32:4:D0;  MCHP_MASTERLINK=MCU_vectorControl_with_fieldWeakening_dsPIC33CK_LVMC_FW_Hurst/BOARD dsPIC33CK LVMC/Microchip Master  MCHP_CRC=4883253  PWMx_PMOD=Complementary  PWM1_HL=PWMxH & PWMxL output enabled  PWM1_swap=off  PWM1H_pol=off  PWM1L_pol=off  PWM2_HL=PWMxH & PWMxL output enabled  PWM2_swap=off  PWM2H_pol=off  PWM2L_pol=off  PWM3_HL=not used  PWM3_swap=off  PWM3H_pol=off  PWM3L_pol=off  PWM4_HL=PWMxH & PWMxL output enabled  PWM4_swap=off  PWM4H_pol=off  PWM4L_pol=off  PWM5_HL=not used  PWM5_swap=off  PWM5H_pol=off  PWM5L_pol=off  PWM6_HL=not used  PWM6_swap=off  PWM6H_pol=off  PWM6L_pol=off  PWM7_HL=not used  PWM7_swap=off  PWM7H_pol=off  PWM7L_pol=off  PWM8_HL=not used  PWM8_swap=off  PWM8H_pol=off  PWM8L_pol=off  PWM9_HL=not used  PWM9_swap=off  PWM9H_pol=off  PWM9L_pol=off  PWM10_HL=not used  PWM10_swap=off  PWM10H_pol=off  PWM10L_pol=off  PWM11_HL=not used  PWM11_swap=off  PWM11H_pol=off  PWM11L_pol=off  PWM12_HL=not used  PWM12_swap=off  PWM12H_pol=off  PWM12L_pol=off  PWM1_ShowTrig=on  PWM1_Init_PGxTRIGABC_s=[0 -1 -1 ]  PWM1_ADTRxEN1=ADC Trigger 1  PWM1_ADTRxEN2=none  PWM1_ADTRxEN3=none  PWM2_ShowTrig=off  PWM2_Init_PGxTRIGABC_s=[-1 -1 -1]  PWM2_ADTRxEN1=none  PWM2_ADTRxEN2=none  PWM2_ADTRxEN3=none  PWM3_ShowTrig=off  PWM3_Init_PGxTRIGABC_s=[-1 -1 -1]  PWM3_ADTRxEN1=none  PWM3_ADTRxEN2=none  PWM3_ADTRxEN3=none  PWM4_ShowTrig=off  PWM4_Init_PGxTRIGABC_s=[-1 -1 -1]  PWM4_ADTRxEN1=none  PWM4_ADTRxEN2=none  PWM4_ADTRxEN3=none  PWM5_ShowTrig=off  PWM5_Init_PGxTRIGABC_s=[-1 -1 -1]  PWM5_ADTRxEN1=none  PWM5_ADTRxEN2=none  PWM5_ADTRxEN3=none  PWM6_ShowTrig=off  PWM6_Init_PGxTRIGABC_s=[-1 -1 -1]  PWM6_ADTRxEN1=none  PWM6_ADTRxEN2=none  PWM6_ADTRxEN3=none  PWM7_ShowTrig=off  PWM7_Init_PGxTRIGABC_s=[-1 -1 -1]  PWM7_ADTRxEN1=none  PWM7_ADTRxEN2=none  PWM7_ADTRxEN3=none  PWM8_ShowTrig=off  PWM8_Init_PGxTRIGABC_s=[-1 -1 -1]  PWM8_ADTRxEN1=none  PWM8_ADTRxEN2=none  PWM8_ADTRxEN3=none  BlockInput_VectorScalar=Vectors (grouped by function)  BlockInput_Period=Not a block input  BlockInput_DutyCycle=a Uint raw input (PWMxmax variable represent max period)  BlockInput_PhaseShift=Not a block input  BlockInput_SEVTCMP=Not a block input  BlockInput_TRIGx=Not a block input  BlockInput_DeadTime=Not a block input  BlockOutput_FaultDisabled=off  BlockOutput_Fault=on  DTC=Positive dead time (ensure period of time with PWM_H and PWM_L disasserted)  FLTSRC1_DTCMP=Dynamic Options  FLTSRC1_DTCMP_TXT=<empty>  FLTSRC2_DTCMP=Dynamic Options  FLTSRC2_DTCMP_TXT=<empty>  FLTSRC3_DTCMP=Dynamic Options  FLTSRC3_DTCMP_TXT=<empty>  FLTSRC4_DTCMP=Dynamic Options  FLTSRC4_DTCMP_TXT=<empty>  FLTSRC5_DTCMP=Dynamic Options  FLTSRC5_DTCMP_TXT=<empty>  FLTSRC6_DTCMP=Dynamic Options  FLTSRC6_DTCMP_TXT=<empty>  FLTSRC7_DTCMP=Dynamic Options  FLTSRC7_DTCMP_TXT=<empty>  FLTSRC8_DTCMP=Dynamic Options  FLTSRC8_DTCMP_TXT=<empty>  FLTSRC9_DTCMP=Dynamic Options  FLTSRC9_DTCMP_TXT=<empty>  FLTSRC10_DTCMP=Dynamic Options  FLTSRC10_DTCMP_TXT=<empty>  FLTSRC11_DTCMP=Dynamic Options  FLTSRC11_DTCMP_TXT=<empty>  FLTSRC12_DTCMP=Dynamic Options  FLTSRC12_DTCMP_TXT=<empty>  DeadTime_s=1e-6  DeadTimeAlt_s=1e-6  DeadTimeComp_s=0  FLTMODx=Disabled  FLTSRCx=Dynamic Options  FLTSRCx_TXT=<empty>  FLTDATx=PWM H/L -> 11  CLMODx=Disabled  CLSRCx=Dynamic Options  CLSRCx_TXT=<empty>  CLDATx=PWM H/L -> 00  FLTLEBENx=off  CLLEBENx=off  LeadEdgeBlkPer_s=5e-7  PHRx=off  PHFx=off  PLRx=off  PLFx=off
      settings: SourceProductName=MPLAB Device Blocks for Simulink
  Port Info : MCHP_Blockset/System Info/Port Info  MCHP_MASTERLINK=MCU_vectorControl_with_fieldWeakening_dsPIC33CK_LVMC_FW_Hurst/BOARD dsPIC33CK LVMC/Microchip Master
      settings: SourceProductName=MPLAB Device Blocks for Simulink
  QEI1 : MCHP_Blockset/QEI/QEI  QEI_REF=1  QEI_MODE=Quadrature Encoder  QEI_x2mode=off  QEI_PulseCountDir=Down  PIN_QEA=Dynamic Options  PIN_QEA_TXT=C12 / P60 / Pin[5]  PIN_QEB=Dynamic Options  PIN_QEB_TXT=C13 / P61 / Pin[6]  SWPAB=on  QEAPOL=off  QEBPOL=off  SampleTime=50e-6  PIN_CCMP=Dynamic Options  PIN_CCMP_TXT=A4 / P20 / Pin[33]  MCHP_PORT={QEI1 A}{QEIA1}5:0:P60;{QEI1 B}{QEIB1}5:0:P61;  MCHP_MASTERLINK=MCU_vectorControl_with_fieldWeakening_dsPIC33CK_LVMC_FW_Hurst/BOARD dsPIC33CK LVMC/Microchip Master  INDXxCNT_Output=is not an output  POSxCNT_Output=is a 16 bits signed block output  RESET_Input=on  PIMOD_mode=position is cyclique between user defined boundaries  PIMOD_modeB=Never reset position  PIMOD_reset=on next INDEX event  PIN_INDEX=Dynamic Options  PIN_INDEX_TXT=C14 / P62 / Pin[7]  IMV=QEA = 0 and QEB = 0  IMV_x2=QEA = 1  PIN_HOME=Dynamic Options  PIN_HOME_TXT=B0 / P32 / Pin[34]  QEIxLEC_GEC=[0 (QEIResolution-1)]  QEIxIC=0  PCIIRQ=off  IDXPOL=on  HOMPOL=on  VELxCNT_Output=is a 16 bits signed block output  INTxHLD_Output=is not an output  MaxPeriod=1e-3  FILTREN=on  QFDIV_popup=Dynamic Options  QFDIV_popup_TXT=4166.67 kHz  FILTER_CutOffFreq=100e3  QEI_IntPri=5
      settings: SourceProductName=MPLAB Device Blocks for Simulink
  Rate Transition3 : RateTransition  Deterministic=off
  SW1 : MCHP_Blockset/Digital IO/Digital Input  PORT=Dynamic Options  PORT_TXT="E   [ 0 : 15 ]"  PIN=11  PACK=off  SIMULTANEOUS=off  ORDERING=None  SampleTime=-1  MCHP_PORT={Digital In}{DIN}2:0:E11;  MCHP_MASTERLINK=MCU_vectorControl_with_fieldWeakening_dsPIC33CK_LVMC_FW_Hurst/BOARD dsPIC33CK LVMC/Microchip Master
      settings: SourceProductName=MPLAB Device Blocks for Simulink
  SW2 : MCHP_Blockset/Digital IO/Digital Input  PORT=Dynamic Options  PORT_TXT="E   [ 0 : 15 ]"  PIN=12  PACK=off  SIMULTANEOUS=off  ORDERING=None  SampleTime=-1  MCHP_PORT={Digital In}{DIN}2:0:E12;  MCHP_MASTERLINK=MCU_vectorControl_with_fieldWeakening_dsPIC33CK_LVMC_FW_Hurst/BOARD dsPIC33CK LVMC/Microchip Master
      settings: SourceProductName=MPLAB Device Blocks for Simulink
  SW3 : MCHP_Blockset/Digital IO/Digital Input  PORT=Dynamic Options  PORT_TXT="E   [ 0 : 15 ]"  PIN=13  PACK=off  SIMULTANEOUS=off  ORDERING=None  SampleTime=-1  MCHP_PORT={Digital In}{DIN}2:0:E13;  MCHP_MASTERLINK=MCU_vectorControl_with_fieldWeakening_dsPIC33CK_LVMC_FW_Hurst/BOARD dsPIC33CK LVMC/Microchip Master
      settings: SourceProductName=MPLAB Device Blocks for Simulink
  Saturation : Saturate  UpperLimit=PWM1max*0.97  LowerLimit=PWM1max*0.03  LinearizeAsGain=off  OutDataTypeStr=uint16
  SinCos : Trigonometry  Operator=sincos  ApproximationMethod=CORDIC
  Timer Info : MCHP_Blockset/System Info/Timer Info  MCHP_MASTERLINK=MCU_vectorControl_with_fieldWeakening_dsPIC33CK_LVMC_FW_Hurst/BOARD dsPIC33CK LVMC/Microchip Master
      settings: SourceProductName=MPLAB Device Blocks for Simulink
  Timing Analysis : Subsystem
  UART Configuration Mikro BUS A - J11 FTDI 2232H UARTb : MCHP_Blockset/BUS UART/UART Configuration  UART_REF=3  BAUD_Choice=Dynamic Options  BAUD_Choice_TXT="3000000         [-0.50%]"  BAUD_Choice_IR=Dynamic Options  BAUD_Choice_IR_TXT=[]  BAUD_Custom=9000000  INT_PRIORITY=0  ALT_IO=on  PIN_RX=Dynamic Options  PIN_RX_TXT=D12 / P76 / Pin[27]  PIN_TX=Dynamic Options  PIN_TX_TXT=D11 / P75 / Pin[36]  MCHP_PORT="{UART3  Rx}{U3RX}3:0:P76;{UART3  Tx}{U3TX}3:0:P75;"  MCHP_MASTERLINK=MCU_vectorControl_with_fieldWeakening_dsPIC33CK_LVMC_FW_Hurst/BOARD dsPIC33CK LVMC/Microchip Master  MCHP_COM_ExtPil=off  TX_IMPLEMENTATION=Circular Buffer  TX_IMPLEMENTATION_default=Circular Buffer  TX_INT_PRIORITY=5  TX_INT_WHEN=has one empty space  TX_INT_WHEN_default=is empty & last char is sent  TX_CIRCULAR_SIZE=1024  TX_DMA_CHANNEL=1  TX_DMA_SIZE=16  TX_TASK_PROTECTION=Delay tasks (default)  TX_INTERRUPT_PROTECTION=Do not send on conflict (default)  TX_INTERRUPT_PROTECTION_default=Do not send on conflict (default)  RX_IMPLEMENTATION=Circular Buffer  RX_IMPLEMENTATION_default=Circular Buffer  RX_INT_PRIORITY=7  RX_INT_WHEN=receive 1 character  RX_CIRCULAR_SIZE=64  RX_DMA_CHANNEL=0  RX_DMA_SIZE=0  DuplexMode=Full duplex (default)  PIN_RX_Inv=off  PIN_TX_Inv=off  PIN_RXTX_Inv=off  ParityBit=No parity (default)  StopBit=1 stop bit (default)  IRDA=off  IdleTime_choice=Dynamic Options  IdleTime_choice_TXT=None  IdleTime_custom=2/50  FlowControl=None  PIN_CTS=Dynamic Options  PIN_CTS_TXT=B0 / P32 / Pin[34]  PIN_RTS=Dynamic Options  PIN_RTS_TXT=B0 / P32 / Pin[34]  PIN_DSR=Dynamic Options  PIN_DSR_TXT=B0 / P32 / Pin[34]  PIN_DTR=Dynamic Options  PIN_DTR_TXT=B0 / P32 / Pin[34]  InitSequence_chkbox=off  BAUD_Choice_InitSeq=Dynamic Options  BAUD_Choice_InitSeq_TXT="110         [+73.40%]"  BAUD_Choice_IR_InitSeq=Dynamic Options  BAUD_Choice_IR_InitSeq_TXT=0  BAUD_Custom_InitSeq=0  InitSequence="uint8(['use VT100 terminal ! ' 13 10 27 'c'  27 '[2J' ] )"
      settings: SourceProductName=MPLAB Device Blocks for Simulink
  UART Configuration Mikro BUS A - J11 Tx-Rx : MCHP_Blockset/BUS UART/UART Configuration  UART_REF=2  BAUD_Choice=Dynamic Options  BAUD_Choice_TXT="8000000         [+0.00%]"  BAUD_Choice_IR=Dynamic Options  BAUD_Choice_IR_TXT=[]  BAUD_Custom=5520000  INT_PRIORITY=0  ALT_IO=on  PIN_RX=Dynamic Options  PIN_RX_TXT=D7 / P71 / Pin[52]  PIN_TX=Dynamic Options  PIN_TX_TXT=C7 / P55 / Pin[40]  MCHP_PORT="{UART2  Rx}{U2RX}3:0:P71;{UART2  Tx}{U2TX}3:0:P55;"  MCHP_MASTERLINK=MCU_vectorControl_with_fieldWeakening_dsPIC33CK_LVMC_FW_Hurst/BOARD dsPIC33CK LVMC/Microchip Master  MCHP_COM_ExtPil=off  TX_IMPLEMENTATION=DMA Circular Buffer  TX_IMPLEMENTATION_default=Circular Buffer  TX_INT_PRIORITY=5  TX_INT_WHEN=is empty & last char is sent  TX_INT_WHEN_default=is empty & last char is sent  TX_CIRCULAR_SIZE=1024  TX_DMA_CHANNEL=2  TX_DMA_SIZE=16  TX_TASK_PROTECTION=Delay tasks (default)  TX_INTERRUPT_PROTECTION=Do not send on conflict (default)  TX_INTERRUPT_PROTECTION_default=Do not send on conflict (default)  RX_IMPLEMENTATION=Circular Buffer  RX_IMPLEMENTATION_default=Circular Buffer  RX_INT_PRIORITY=7  RX_INT_WHEN=receive 1 character  RX_CIRCULAR_SIZE=64  RX_DMA_CHANNEL=0  RX_DMA_SIZE=0  DuplexMode=Full duplex (default)  PIN_RX_Inv=off  PIN_TX_Inv=off  PIN_RXTX_Inv=off  ParityBit=No parity (default)  StopBit=1 stop bit (default)  IRDA=off  IdleTime_choice=Dynamic Options  IdleTime_choice_TXT=None  IdleTime_custom=2/50  FlowControl=None  PIN_CTS=Dynamic Options  PIN_CTS_TXT=B0 / P32 / Pin[34]  PIN_RTS=Dynamic Options  PIN_RTS_TXT=B0 / P32 / Pin[34]  PIN_DSR=Dynamic Options  PIN_DSR_TXT=B0 / P32 / Pin[34]  PIN_DTR=Dynamic Options  PIN_DTR_TXT=B0 / P32 / Pin[34]  InitSequence_chkbox=off  BAUD_Choice_InitSeq=Dynamic Options  BAUD_Choice_InitSeq_TXT="110         [+73.40%]"  BAUD_Choice_IR_InitSeq=Dynamic Options  BAUD_Choice_IR_InitSeq_TXT=0  BAUD_Custom_InitSeq=0  InitSequence="uint8(['use VT100 terminal ! ' 13 10 27 'c'  27 '[2J' ] )"
      settings: SourceProductName=MPLAB Device Blocks for Simulink
  UART Configuration Mikro BUS B - J12 : MCHP_Blockset/BUS UART/UART Configuration  Commented=on  UART_REF=3  BAUD_Choice=Dynamic Options  BAUD_Choice_TXT="8000000         [+0.00%]"  BAUD_Choice_IR=Dynamic Options  BAUD_Choice_IR_TXT=[]  BAUD_Custom=9000000  INT_PRIORITY=0  ALT_IO=on  PIN_RX=Dynamic Options  PIN_RX_TXT=D5 / P69 / Pin[54]  PIN_TX=Dynamic Options  PIN_TX_TXT=D6 / P70 / Pin[53]  MCHP_PORT="{UART3  Tx}{U3TX}3:0:P70;"  MCHP_MASTERLINK=MCU_vectorControl_with_fieldWeakening_dsPIC33CK_LVMC_FW_Hurst/BOARD dsPIC33CK LVMC/Microchip Master  MCHP_COM_ExtPil=off  TX_IMPLEMENTATION=Circular Buffer  TX_IMPLEMENTATION_default=Circular Buffer  TX_INT_PRIORITY=4  TX_INT_WHEN=has one empty space  TX_INT_WHEN_default=is empty & last char is sent  TX_CIRCULAR_SIZE=256  TX_DMA_CHANNEL=2  TX_DMA_SIZE=16  TX_TASK_PROTECTION=Delay tasks (default)  TX_INTERRUPT_PROTECTION=Do not send on conflict (default)  TX_INTERRUPT_PROTECTION_default=Do not send on conflict (default)  RX_IMPLEMENTATION=Do not implement Rx  RX_IMPLEMENTATION_default=Circular Buffer  RX_INT_PRIORITY=7  RX_INT_WHEN=receive 1 character  RX_CIRCULAR_SIZE=64  RX_DMA_CHANNEL=0  RX_DMA_SIZE=0  DuplexMode=Full duplex (default)  PIN_RX_Inv=off  PIN_TX_Inv=off  PIN_RXTX_Inv=off  ParityBit=No parity (default)  StopBit=1 stop bit (default)  IRDA=off  IdleTime_choice=Dynamic Options  IdleTime_choice_TXT=None  IdleTime_custom=2/50  FlowControl=None  PIN_CTS=Dynamic Options  PIN_CTS_TXT=B0 / P32 / Pin[34]  PIN_RTS=Dynamic Options  PIN_RTS_TXT=B0 / P32 / Pin[34]  PIN_DSR=Dynamic Options  PIN_DSR_TXT=B0 / P32 / Pin[34]  PIN_DTR=Dynamic Options  PIN_DTR_TXT=B0 / P32 / Pin[34]  InitSequence_chkbox=off  BAUD_Choice_InitSeq=Dynamic Options  BAUD_Choice_InitSeq_TXT="110         [+73.40%]"  BAUD_Choice_IR_InitSeq=Dynamic Options  BAUD_Choice_IR_InitSeq_TXT=0  BAUD_Custom_InitSeq=0  InitSequence="uint8(['use VT100 terminal ! ' 13 10 27 'c'  27 '[2J' ] )"
      settings: SourceProductName=MPLAB Device Blocks for Simulink
  UART configuration USB - J6 PKOB - J13 : MCHP_Blockset/BUS UART/UART Configuration  UART_REF=1  BAUD_Choice=Dynamic Options  BAUD_Choice_TXT="460800         [+0.01%]"  BAUD_Choice_IR=Dynamic Options  BAUD_Choice_IR_TXT=[]  BAUD_Custom=115200  INT_PRIORITY=0  ALT_IO=on  PIN_RX=Dynamic Options  PIN_RX_TXT=D14 / P78 / Pin[13]  PIN_TX=Dynamic Options  PIN_TX_TXT=D13 / P77 / Pin[14]  MCHP_PORT="{UART1  Rx}{U1RX}3:0:P78;{UART1  Tx}{U1TX}3:0:P77;"  MCHP_MASTERLINK=MCU_vectorControl_with_fieldWeakening_dsPIC33CK_LVMC_FW_Hurst/BOARD dsPIC33CK LVMC/Microchip Master  MCHP_COM_ExtPil=off  TX_IMPLEMENTATION=DMA Circular Buffer  TX_IMPLEMENTATION_default=Circular Buffer  TX_INT_PRIORITY=5  TX_INT_WHEN=is empty  TX_INT_WHEN_default=is empty & last char is sent  TX_CIRCULAR_SIZE=256  TX_DMA_CHANNEL="0   (Lowest Priority)"  TX_DMA_SIZE=512  TX_TASK_PROTECTION=Delay tasks (default)  TX_INTERRUPT_PROTECTION=Do not send on conflict (default)  TX_INTERRUPT_PROTECTION_default=Do not send on conflict (default)  RX_IMPLEMENTATION=Circular Buffer  RX_IMPLEMENTATION_default=Circular Buffer  RX_INT_PRIORITY=7  RX_INT_WHEN=receive 1 character  RX_CIRCULAR_SIZE=64  RX_DMA_CHANNEL=0  RX_DMA_SIZE=0  DuplexMode=Full duplex (default)  PIN_RX_Inv=off  PIN_TX_Inv=off  PIN_RXTX_Inv=off  ParityBit=No parity (default)  StopBit=1 stop bit (default)  IRDA=off  IdleTime_choice=Dynamic Options  IdleTime_choice_TXT=None  IdleTime_custom=2/50  FlowControl=None  PIN_CTS=Dynamic Options  PIN_CTS_TXT=B0 / P32 / Pin[34]  PIN_RTS=Dynamic Options  PIN_RTS_TXT=B0 / P32 / Pin[34]  PIN_DSR=Dynamic Options  PIN_DSR_TXT=B0 / P32 / Pin[34]  PIN_DTR=Dynamic Options  PIN_DTR_TXT=B0 / P32 / Pin[34]  InitSequence_chkbox=off  BAUD_Choice_InitSeq=Dynamic Options  BAUD_Choice_InitSeq_TXT="115200         [+0.01%]"  BAUD_Choice_IR_InitSeq=Dynamic Options  BAUD_Choice_IR_InitSeq_TXT=0  BAUD_Custom_InitSeq=0  InitSequence="uint8(['use VT100 terminal ! ' 13 10 27 'c'  27 '[2J' ] )"
      settings: SourceProductName=MPLAB Device Blocks for Simulink
  Weighted Sample Time : SampleTimeMath  TsampMathOp=/  weightValue=QEIResolution / (2*pi)  OutDataTypeStr=Inherit: Inherit via back propagation
  electrical position : Gain  Gain=n/QEIResolution  OutDataTypeStr=fixdt(0,16,16)
  fract range: 0-21V : DataTypeConversion  OutDataTypeStr=fixdt(0,16,3.3/65536*21,0)  ConvertRealWorld=Stored Integer (SI)
  mechanical position : Gain  Gain=1/QEIResolution  OutDataTypeStr=fixdt(0,16,16)
  per_unit : Subsystem
  range: +- 21.83A : DataTypeConversion  OutDataTypeStr=fixdt(1,16,21.83/32768,0)  ConvertRealWorld=Stored Integer (SI)
  range: +- 21.83A1 : DataTypeConversion  OutDataTypeStr=fixdt(1,16,21.83/32768,0)  ConvertRealWorld=Stored Integer (SI)
  to rad : Gain  Gain=2*pi  OutDataTypeStr=fixdt(0,16,13)
  unitary : DataTypeConversion  OutDataTypeStr=fixdt(0,16,16)  ConvertRealWorld=Stored Integer (SI)
  sensors : Outport  VectorParamsAs1DForOutWhenUnconnected=on
  wires:
  ADC/4(pot) -> Downsample x20/1(In1)
  SW3/1 -> Bus Creator/3  "BTN 3"
  LED 2/1 -> LED_2/1
  SW2/1 -> Bus Creator/2  "BTN 2"
  QEI1/1 -> Bus Creator7/2, mechanical position/1, electrical position/1  "theta_RAW"
  Mux/1 -> Bus Creator6/3  "SinCos_th"
  mechanical position/1 -> Encoder Offset_/1
  ADC/5(V_BUS) -> Downsample x20 _/1(In1)
  Downsample x20/1(Out1) -> unitary/1
  SinCos/1 -> Mux/1
  Saturation/1 -> PWM_HS_FEP/1
  Bus Creator2/1 -> Bus Creator5/1  "MCU"
  ADC/1(Ia) -> Mux1/1
  Bus Creator4/1 -> Bus Creator5/5  "optical coder"
  Bus Creator/1 -> Bus Creator5/2  "BTN"
  SinCos/2 -> Mux/2
  Downsample Averaged x20/1(Out1) -> Bus Creator3/3  "omega_m_rad"
  to rad/1 -> SinCos/1
  SW1/1 -> Bus Creator/1  "BTN 1"
  PWM Scaling/1(PWM) -> Saturation/1
  electrical position/1 -> Encoder Offset/1
  Weighted Sample Time/1 -> Data Type Duplicate/2, Downsample Averaged x20/1(In1)
  Timing Analysis/2(CPU Overload) -> Bus Creator2/2  "overload"
  Timing Analysis/1(CPU Load) -> Bus Creator2/1  "load"
  QEI1/2 -> Data Type Duplicate/1, Bus Creator7/1, Weighted Sample Time/1  "omega_RAW"
  range: +- 21.83A/1 -> Bus Creator1/1  "I_ab"
  fract range: 0-21V/1 -> Bus Creator1/4  "V_bus"
  Bus Creator1/1 -> Bus Creator5/3  "ADC"
  INIT/1 -> Data Type Conversion4/1
  ADC/3(IBus) -> range: +- 21.83A1/1, per_unit/3(I_bus)
  ADC/2(Ib) -> Mux1/2
  Bus Creator5/1 -> sensors/1
  PWM [0 1]/1 -> PWM Scaling/1(vabc [0 1])
  Bus Creator3/1 -> Bus Creator4/2  "mecc"
  Bus Creator6/1 -> Bus Creator4/1  "elec"
  LED 1/1 -> LED_1/1
  reset encoder/1 -> QEI1/1
  per_unit/1(ADC_unit) -> Bus Creator5/4  "ADC_unit"
  Data Type Conversion2/1 -> Bus Creator6/1  "theta_e_rad"
  Bus Creator7/1 -> Bus Creator4/3  "RAW"
  range: +- 21.83A1/1 -> Bus Creator1/2  "I_bus"
  unitary/1 -> per_unit/1(pot), Bus Creator1/3  "pot"
  Downsample x20 _/1(Out1) -> per_unit/4(V_bus), fract range: 0-21V/1
  Center & sign reversal/1(Iab) -> range: +- 21.83A/1, per_unit/2(I_ab)
  Rate Transition3/1 -> Center & sign reversal/2(Bias Update)
  Mux1/1 -> Center & sign reversal/1(I_ab)
  Data Type Conversion3/1 -> Bus Creator3/1  "theta_m_rad"
  Encoder Offset/1 -> Bus Creator6/2, Data Type Conversion2/1, to rad/1  "theta_e_unit"
  Encoder Offset_/1 -> Bus Creator3/2, Data Type Conversion3/1  "theta_m_unit"
  Data Type Conversion4/1 -> Rate Transition3/1
